simulink model "dampedSpring"  (Simulink 4.00)
settings: Solver=ode45  StartTime=0.0  StopTime=0.0001  RelTol=1e-3
settings Model: LastModifiedBy=JimmyL

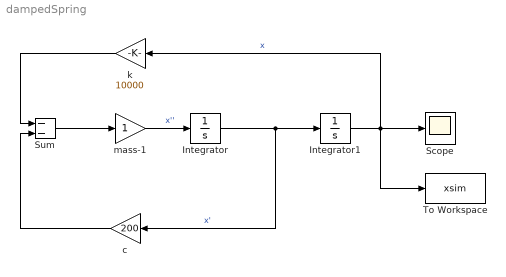
== system dampedSpring ==
  Integrator : Integrator  ExternalReset=none  InitialConditionSource=internal  InitialCondition=0  LimitOutput=off  UpperSaturationLimit=inf  LowerSaturationLimit=-inf  ShowSaturationPort=off  ShowStatePort=off  AbsoluteTolerance=auto
  Integrator1 : Integrator  ExternalReset=none  InitialConditionSource=internal  InitialCondition=0.01  LimitOutput=off  UpperSaturationLimit=inf  LowerSaturationLimit=-inf  ShowSaturationPort=off  ShowStatePort=off  AbsoluteTolerance=auto
  Scope : Scope
      settings: TimeRange=0.1  YMin=-0.02  YMax=0.1  SaveToWorkspace=off  SaveName=ScopeData  LimitDataPoints=on  MaxDataPoints=5000  Decimation=0.1  SampleInput=on  SampleTime=1e-4
  Sum : Sum  Inputs=--  SaturateOnIntegerOverflow=on
  To Workspace : ToWorkspace  VariableName=xsim  SampleTime=1e-9  SaveFormat=Array
  c : Gain  Orientation=left  Gain=200  Multiplication=Element-wise(K.*u)  SaturateOnIntegerOverflow=on
  k : Gain  Orientation=left  Gain=10000  Multiplication=Element-wise(K.*u)  SaturateOnIntegerOverflow=on
  mass-1 : Gain  Gain=1  Multiplication=Element-wise(K.*u)  SaturateOnIntegerOverflow=on
  wires:
  Sum/1 -> mass-1/1
  mass-1/1 -> Integrator/1  "x''"
  c/1 -> Sum/2
  Integrator/1 -> Integrator1/1, c/1  "x'"
  k/1 -> Sum/1
  Integrator1/1 -> k/1, Scope/1, To Workspace/1  "x"
